simulink library "mbed_lib_hk"  (R2015a)
settings: Solver=ode45  SolverMode=SingleTasking  StartTime=0.0  StopTime=10.0  RelTol=1e-3
undefined symbols (not defined in the file): A
libraries: mbed_lib x1
(part 1 of 2)
settings Model: CovSFcnEnable=off  Creator=syoon  LastModifiedBy=Hendrik
settings OptimizationCC: BlockReduction=off  BooleanDataType=off
settings DebuggingCC: SaveWithParameterizedLinksMsg=none  UnderspecifiedInitializationDetection=Classic  MergeDetectMultiDrivingBlocksExec=none  SignalResolutionControl=TryResolveAllWithWarning  StrictBusMsg=Warning
settings HardwareCC: TargetUnknown=on

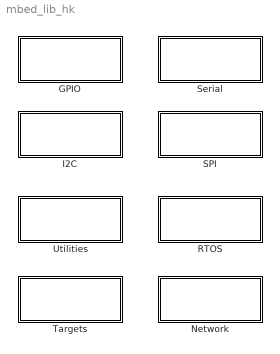
== system mbed_lib_hk ==
  GPIO : Subsystem
      mask Display: disp('GPIO')
  I2C : Subsystem
      mask Display: disp('I2C')
  Network : Subsystem
      mask Display: disp('Network')
  RTOS : Subsystem
      mask Display: disp('RTOS')
  SPI : Subsystem
      mask Display: disp('SPI')
  Serial : Subsystem
      mask Display: disp('Serial')
  Targets : Subsystem
      settings: OpenFcn=mbed_targets
      mask Display: disp('Targets')
  Utilities : Subsystem
      mask Display: disp('Utilities')

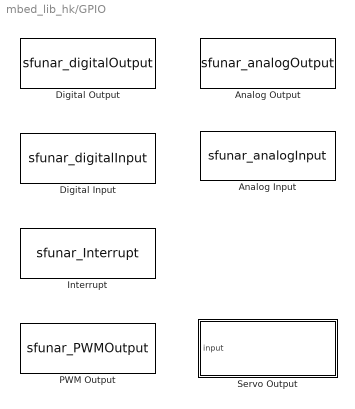
== system mbed_lib_hk/GPIO ==
  Analog Input : S-Function  FunctionName=sfunar_analogInput  Parameters=uint8(SParameter1), SampleTime, uint8(SParameter2)  mask(mbed Analog Input){SParameter2=A, SParameter1=0, SampleTime=-1}
      mask prompts: SParameter2 "Port Name:"; SParameter1 "Pin Number:"; SampleTime "Sample time (-1 for inherited):"
      mask help:
      | Reads the analog voltage input from the specified pin.
      |
      | The range of input on the pin is between 0 and Vref corresponding to a block output of 0 to 1.0f (in %) or 0 to 1024/4096/.. .
      mask Help:
      | <p>This block calls the AnalogIn.read() and AnalogIn.read_u16() function from the mbed library.
      | <p>For more information see: <a href="http://mbed.org ...">Arduino - AnalogRead</a>
      mask TypeOptions SParameter2: A | B | C | D | E | F | G | H | I | J | K
      mask TypeOptions SParameter1: 0 | 1 | 2 | 3 | 4 | 5 | 6 | 7 | 8 | 9 | 10 | 11 | 12 | 13 | 14 | 15
      mask Display:
      | offset=0.0;
      | plot([0+offset:0.025:0.25+offset],0.3*sin(2*pi*[0:0.1:1])+0.5)
      | disp(['Pin ', SParameter2+64, '.', num2str(SParameter1-1)]);
      | port_label('output',1,'RAW');
      | port_label('output',2,'0-1.0f');
  Analog Output : S-Function  FunctionName=sfunar_analogOutput  Parameters=uint8(SParameter1), SampleTime, uint8(SParameter2), uint8(inputVariant)  mask(mbed Analog Output){SParameter2=A, SParameter1=0, inputVariant=Double: 0 - 1.0f, SampleTime=-1}
      mask prompts: SParameter2 "Port Name:"; SParameter1 "Pin Number:"; inputVariant "Input data format"; SampleTime "Sample time (-1 for inherited):"
      mask help:
      | Writes an analog voltage output to the specified pin using the integrated DAC.
      |
      | The input to this block is a float between 0 and 1.0 (in %) or an integer between 0 and 1024/4096/.. corresponding to an output voltage between 0 to Vref.
      mask Help:
      | <p>This block calls the analogWrite() function from the Arduino language library.
      | <p>For more information see: <a href="http://arduino.cc/en/Reference/AnalogWrite">Arduino - AnalogWrite</a>
      mask TypeOptions SParameter2: A | B | C | D | E | F | G | H | I | J | K
      mask TypeOptions SParameter1: 0 | 1 | 2 | 3 | 4 | 5 | 6 | 7 | 8 | 9 | 10 | 11 | 12 | 13 | 14 | 15
      mask TypeOptions inputVariant: Uint16: RAW (0x0YYY) | Double: 0 - 1.0f
      mask Display:
      | offset=0.7;
      | plot([0+offset:0.025:0.25+offset],0.3*sin(2*pi*[0:0.1:1])+0.5)
      | disp(['Pin ', SParameter2+64, '.', num2str(SParameter1-1)]);
      | p={'RAW'; '0-1.0f'};
      | port_label('input',1,p{inputVariant});
  Digital Input : S-Function  FunctionName=sfunar_digitalInput  Parameters=uint8(SParameter1), SampleTime, uint8(SParameter2), uint8(SParameter3)  mask(mbed Digital Input){SParameter2=A, SParameter1=0, SParameter3=PullDefault, SampleTime=-1}
      mask prompts: SParameter2 "Port Name"; SParameter1 "Pin Number:"; SParameter3 "Input Mode"; SampleTime "Sample time (-1 for inherited):"
      mask help:
      | Reads the digital value from the specified pin.
      |
      | The block outputs 1 for high and 0 for low.
      mask Help:
      | <p>This block uses the DigitalIn api of the mbed library.
      | <p>For more information see: <a href="http://arduino.cc/en/Reference/DigitalRead">Arduino - DigitalRead</a>
      mask TypeOptions SParameter2: A | B | C | D | E | F | G | H | I | J | K
      mask TypeOptions SParameter1: 0 | 1 | 2 | 3 | 4 | 5 | 6 | 7 | 8 | 9 | 10 | 11 | 12 | 13 | 14 | 15
      mask TypeOptions SParameter3: PullDefault | PullUp | PullDown | PullNone
      mask Display:
      | plot([0 0.15 0.15 0.35 0.35 0.5],[0.3 0.3 0.7 0.7 0.3 0.3])
      | port_label('output',1,['Pin ', SParameter2+64, '.', num2str(SParameter1-1)]);
  Digital Output : S-Function  FunctionName=sfunar_digitalOutput  Parameters=uint8(SParameter1), SampleTime, uint8(SParameter2), uint8(SParameter3)  mask(mbed Digital Output){SParameter2=A, SParameter1=0, SParameter3=PullDefault, SampleTime=-1}
      mask prompts: SParameter2 "Port Name:"; SParameter1 "Pin Number:"; SParameter3 "Output Mode"; SampleTime "Sample time (-1 for inherited):"
      mask help:
      | Sends the digital value to the specified port.pin.
      | The pin can be configured as push-pull (pp) or open drain output (od).
      |
      | An input of 1 sets the pin high and 0 sets the pin low.
      mask Help:
      | <p>This block uses the DigitalOut class of the mbed library.
      | <p>For more information see: <a href="http://mbed.org">mbed - DigitalWrite</a>
      mask TypeOptions SParameter2: A | B | C | D | E | F | G | H | I | J | K
      mask TypeOptions SParameter1: 0 | 1 | 2 | 3 | 4 | 5 | 6 | 7 | 8 | 9 | 10 | 11 | 12 | 13 | 14 | 15
      mask TypeOptions SParameter3: PullDefault | PullUp | PullDown | PullNone | Repeater | OpenDrain
      mask Display:
      | plot([0.5 0.65 0.65 0.85 0.85 1],[0.3 0.3 0.7 0.7 0.3 0.3])
      | port_label('input',1,['Pin ', SParameter2+64, '.', num2str(SParameter1-1)]);
  Interrupt : S-Function  FunctionName=sfunar_Interrupt  Parameters=uint8(PortName), uint8(PinName), uint8(Interrupt)  mask{PortName=A, PinName=0, Interrupt=None}
      mask prompts: PortName "Port Name"; PinName "Pin Name"
      mask TypeOptions PortName: A | B | C | D | E | F | G | H | I | J | K
      mask TypeOptions PinName: 0 | 1 | 2 | 3 | 4 | 5 | 6 | 7 | 8 | 9 | 10 | 11 | 12 | 13 | 14 | 15
      mask TypeOptions Interrupt: None | Rise | Fall | Both
      mask Display:
      | p={'None'; 'Rise'; 'Fall'; 'Both'};
      | disp(['Interrupt: ' p{Interrupt} ' Pin ', PortName+64, '.', num2str(PinName-1)]);
  PWM Output : S-Function  FunctionName=sfunar_PWMOutput  Parameters=SampleTime, uint8(SParameter1), uint8(SParameter2), uint32(SParameter3)  mask(mbed PWM Output){SParameter1=A, SParameter2=0, SParameter3=1000, SampleTime=-1}
      mask prompts: SParameter1 "PWM Port:"; SParameter2 "PWM Pin:"; SParameter3 "Period (µs):"; SampleTime "Sample time (-1 for inherited):"
      mask help:
      | Creates an pwm output signal on the specified pin using a configurable PWM period.
      |
      | The input to this block is a float between 0.0f and 1.0f corresponding to 0 to 100% pulsewidth.
      mask Help:
      | <p>This block calls the analogWrite() function from the Arduino language library.
      | <p>For more information see: <a href="http://arduino.cc/en/Reference/AnalogWrite">Arduino - AnalogWrite</a>
      mask TypeOptions SParameter1: A | B | C | D | E | F | G | H | I | J | K
      mask TypeOptions SParameter2: 0 | 1 | 2 | 3 | 4 | 5 | 6 | 7 | 8 | 9 | 10 | 11 | 12 | 13 | 14 | 15
      mask Display:
      | plot([0.5 0.65 0.65 0.85 ],[0.3 0.3 0.7 0.7 ])
      | plot([0.8 0.8],[0.7 0.3])
      | plot([0.825 0.825],[0.7 0.3])
      | plot([0.85 0.85],[0.7 0.3])
      | plot([0.8 1],[0.3 0.3])
      | disp(['Pin ' SParameter1+64 '.' num2str(SParameter2-1)]);
      | port_label('input',1,'0-1.0f');
  Servo Output : Subsystem  mask{SParameter1=A, SParameter2=0, PW_min=1, PW_max=2}
      mask prompts: SParameter1 "PWM Port:"; SParameter2 "PWM Pin:"; PW_min "PW min (ms)"; PW_max "PW max (ms)"
      mask help:
      | Block generates PWM signal with 50Hz period for control of standard RC-servo.
      | Minimum and maximum pulsewidth can be configured.
      | Input is a double value between 0 and 1.0
      mask TypeOptions SParameter1: PWM Output/SParameter1
      mask TypeOptions SParameter2: PWM Output/SParameter2
      mask Display:
      | disp('Servo Output\n');
      | disp(['\nPin ' SParameter1+64 '.' num2str(SParameter2-1) ]);
      | port_label('input',1,'0-1.0f');

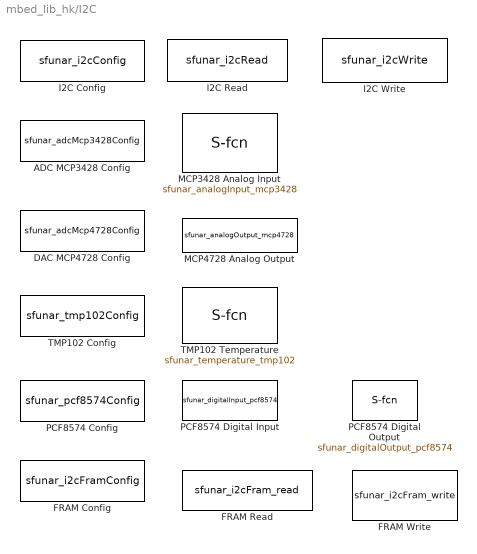
== system mbed_lib_hk/I2C ==
  ADC MCP3428 Config : S-Function  Priority=1  FunctionName=sfunar_adcMcp3428Config  Parameters=uint8(SParameter1)  mask(MCP3428 Configuration){SParameter1=0}
      mask prompts: SParameter1 "Device Sub Address"
      mask help:
      | This blocks sets up the MCP3428 on the I2C board. You must have one of these blocks in any model that ues this device.
      |
      | The sub-address must match the pin configuration on the board. See the board documentation for details.
      mask Display: disp(['Sub-Address: ' num2str(SParameter1) ]);
  DAC MCP4728 Config : S-Function  Priority=1  FunctionName=sfunar_adcMcp4728Config  Parameters=uint8(SParameter1)  mask(MCP4728 Configuration){SParameter1=0}
      mask prompts: SParameter1 "Device Sub Address"
      mask help:
      | This blocks sets up the MCP4728 on the I2C board. You must have one of these blocks in any model that ues this device.
      |
      | The sub-address must match the pin configuration on the board. See the board documentation for details.
      mask Display: disp(['Sub-Address: ' num2str(SParameter1) ]);
  FRAM Config : S-Function  Priority=1  FunctionName=sfunar_i2cFramConfig  mask(I2C Fram Config){}
  FRAM Read : S-Function  FunctionName=sfunar_i2cFram_read  Parameters=uint8(SParameter1-1), SampleTime, boolean(errEn)  mask(Fram Read){SampleTime=-1, SParameter1=on startup, errEn=on}
      mask prompts: SampleTime "Sample time (-1 for inherited):"; SParameter1 "Read condition"; errEn "Enable error output port"
      mask help: Reads one byte from the FRAM.
      mask TypeOptions SParameter1: on startup | on each step
      mask Display:
      | port_label('input', 1, 'Page Address');
      | port_label('input', 2, 'Word Address');
      | 
      | port_label('output',1,'Value');
      | if errEn
      | port_label('output',2,'Error');
      | end
  FRAM Write : S-Function  FunctionName=sfunar_i2cFram_write  Parameters=uint8(SParameter1-1), SampleTime, boolean(errEn)  mask(FRAM Write){SampleTime=-1, SParameter1=on startup, errEn=on}
      mask prompts: SampleTime "Sample time (-1 for inherited):"; SParameter1 "Write condition"; errEn "Enable error output port"
      mask help: Writes one byte to the FRAM
      mask TypeOptions SParameter1: on startup | on each step
      mask Display:
      | port_label('input', 1, 'Page Address');
      | port_label('input', 2, 'Word Address');
      | port_label('input', 3, 'Data');
      | 
      | if errEn
      | port_label('output',1,'Error');
      | end
  I2C Config : S-Function  Priority=0  FunctionName=sfunar_i2cConfig  Parameters=uint8(0), uint8(SParameter2), uint8(SParameter3), uint8(SParameter4), uint8(SParameter5), SParameter6, uint8(I2cPort)  mask(I2C Configuration){I2cPort=1, SParameter6=100000, SParameter2=B, SParameter3=9, SParameter4=B, SParameter5=8}
      mask prompts: I2cPort "I2C Port"; SParameter6 "Bus frequency: [Hz]"; SParameter2 "Port Name (SDA)"; SParameter3 "Pin Number (1-16):"; SParameter4 "Port Name (SCL)"; SParameter5 "Pin Number (1-16):"
      mask help: This blocks sets up the I2C connection on the mbed board. You must have one of these blocks in any model that ues I2C blocks.
      mask TypeOptions I2cPort: 1 | 2 | 3
      mask TypeOptions SParameter2: A | B | C | D | E | F
      mask TypeOptions SParameter3: 0 | 1 | 2 | 3 | 4 | 5 | 6 | 7 | 8 | 9 | 10 | 11 | 12 | 13 | 14 | 15
      mask TypeOptions SParameter4: A | B | C | D | E | F
      mask TypeOptions SParameter5: 0 | 1 | 2 | 3 | 4 | 5 | 6 | 7 | 8 | 9 | 10 | 11 | 12 | 13 | 14 | 15
      mask Display:
      | disp(['I2C ' num2str(I2cPort) '\n\n']);
      | disp(['SDA: ' SParameter2+64 '.' num2str(SParameter3-1) ', SCL: ' SParameter4+64, '.' num2str(SParameter5-1)]);
      | disp(['\n\nFrequency: ' num2str(SParameter6) ' HZ']);
  I2C Read : S-Function  FunctionName=sfunar_i2cRead  Parameters=SampleTime, boolean(AddressFlag), uint8(SlaveAddress), boolean(ByteCountFlag), uint8(NumBytes), boolean(Repeated), uint8(I2cPort)  mask{I2cPort=1, AddressFlag=off, SlaveAddress=0, ByteCountFlag=off, NumBytes=1, Repeated=off, SampleTime=-1}
      mask prompts: I2cPort "I2C Port:"; AddressFlag "external address input"; SlaveAddress "Slave address (7 bit):"; ByteCountFlag "external byte count"; NumBytes "Number of bytes to read:"; SampleTime "Sample time (-1 for inherited):"
      mask TypeOptions I2cPort: 1 | 2 | 3
      mask Display:
      | disp(['I2C ' num2str(I2cPort) '\n']);
      | if AddressFlag == 0
      |     disp(['\nAddress: 0x' dec2hex(SlaveAddress)]);
      | else
      |    disp(['\nAddress: external']);
      |    port_label('input',1,'addr');
      | end
      | 
      | if ByteCountFlag == 1 && AddressFlag == 0
      |     port_label('input',1,'cnt');
      | elseif ByteCountFlag == 1 && AddressFlag == 1
      |     port_label('input',2,'cnt');
      | end
  I2C Write : S-Function  FunctionName=sfunar_i2cWrite  Parameters=SampleTime, boolean(AddressFlag), uint8(SlaveAddress), boolean(ByteCountFlag), boolean(Repeated), uint8(I2cPort)  mask{I2cPort=1, AddressFlag=off, SlaveAddress=0, ByteCountFlag=off, Repeated=off, SampleTime=-1}
      mask prompts: I2cPort "I2C Port:"; AddressFlag "external address input"; SlaveAddress "Slave address (7bit):"; ByteCountFlag "external byte count"; SampleTime "Sample time (-1 for inherited):"
      mask TypeOptions I2cPort: 1 | 2 | 3
      mask Display:
      | disp(['I2C ' num2str(I2cPort) '\n']);
      | 
      | port_label('input', 1, 'data');
      | 
      | if AddressFlag == 1
      |     disp(['\nAddress: external']);
      |     port_label('input', 2, 'addr');
      | else
      |     disp(['\nAddress: 0x' dec2hex(SlaveAddress)]);
      | end
      | 
      | if AddressFlag == 0 && ByteCountFlag == 1
      |     port_label('input', 2, 'cnt');
      | elseif AddressFlag == 1 && ByteCountFlag == 1
      |     port_label('input', 3, 'cnt');
      | end
  MCP3428 Analog Input : S-Function  FunctionName=sfunar_analogInput_mcp3428  Parameters=uint8(SParameter1-1), SampleTime, uint8(SParameter2), uint8(SParameter3), boolean(ErrorOutputEnable)  mask(MCP3428 Analog Input){SampleTime=-1, SParameter1=0, SParameter2=240 SPS (12 bit), SParameter3=1X, ErrorOutputEnable=on}
      mask prompts: SampleTime "Sample time (-1 for inherited):"; SParameter1 "Pin Number:"; SParameter2 "Sample-Rate"; SParameter3 "PGA-Gain"; ErrorOutputEnable "Enable error output port"
      mask help:
      | Reads the analog voltage input from the specified pin on the MCP3428.
      |
      | Warning: This block waits for a complete conversation during the execution step.
      | If the sample time is too small it will have an impact on the step time of the whole model!
      mask TypeOptions SParameter1: 0 | 1 | 2 | 3 | 4 | 5 | 6 | 7
      mask TypeOptions SParameter2: 240 SPS (12 bit) | 60 SPS (14 bit) | 15 SPS (16 bit)
      mask TypeOptions SParameter3: 1X | 2X | 4X | 8X
      mask Display:
      | plot([0:0.01:0.25],0.3*sin(2*pi*[0:0.04:1])+0.5)
      | disp(['Pin ', num2str(SParameter1-1)]);
      | port_label('output',1,'RAW');
      | port_label('output',2,'V');
      | port_label('output',3,'0-1');
      | if ErrorOutputEnable
      |     port_label('output',4,'Error');
      | end
  MCP4728 Analog Output : S-Function  FunctionName=sfunar_analogOutput_mcp4728  Parameters=uint8(SParameter1-1), SampleTime, boolean(errEn), uint8(inputVariant-1), boolean(internalRef-1), boolean(gain2x-1)  mask(MCP4728 Analog Output){SampleTime=-1, SParameter1=0, inputVariant=Uint16: right aligned (0x0YYY), internalRef=VDD (3.3 V), gain2x=1X, errEn=on}
      mask prompts: SampleTime "Sample time (-1 for inherited):"; SParameter1 "Pin Number:"; inputVariant "Input data format"; internalRef "Reference voltage"; gain2x "Gain"; errEn "Enable error output port"
      mask help: Approximates an analog output on the specified pin on the MCP4728.
      mask TypeOptions SParameter1: 0 | 1 | 2 | 3
      mask TypeOptions inputVariant: Uint16: right aligned (0x0YYY) | Uint16: left aligned (0xYYY0) | Double: Voltage in V | Double: 0 ... 1
      mask TypeOptions internalRef: VDD (3.3 V) | Internal (2.048 V)
      mask TypeOptions gain2x: 1X | 2X (only for internal VRef)
      mask Display:
      | plot([0.5-.125:0.01:0.75-.125],0.3*sin(2*pi*[0:0.04:1])+0.5)
      | port_label('input',1,['Pin ', num2str(SParameter1-1)]);
      | if errEn
      |     port_label('output',1,'Error');
      | end
  PCF8574 Config : S-Function  Priority=1  FunctionName=sfunar_pcf8574Config  Parameters=uint8(SParameter1)  mask(PCF8574 Configuration){SParameter1=0}
      mask prompts: SParameter1 "Device Sub Address"
      mask help:
      | This blocks sets up the PCF8574 on the I2C board. You must have one of these blocks in any model that ues this device.
      |
      | The sub-address must match the pin configuration on the board. See the board documentation for details.
      mask Display: disp(['Sub-Address: ' num2str(SParameter1) ]);
  PCF8574 Digital Input : S-Function  FunctionName=sfunar_digitalInput_pcf8574  Parameters=uint8(SParameter1-1), SampleTime, boolean(errEn)  mask(PCF8574 Digital Input){SampleTime=-1, SParameter1=0, errEn=on}
      mask prompts: SampleTime "Sample time (-1 for inherited):"; SParameter1 "Pin Number:"; errEn "Enable error output port"
      mask help:
      | Reads the digital value from the specified pin of the PCF8574.
      |
      | Note: The PCF8574 has an pull up current source on each pin.
      mask TypeOptions SParameter1: 0 | 1 | 2 | 3 | 4 | 5 | 6 | 7
      mask Display:
      | disp(['Pin ', num2str(SParameter1-1)]);
      | port_label('output',1,'Value');
      | if errEn
      | port_label('output',2,'Error');
      | end
  PCF8574 Digital Output : S-Function  FunctionName=sfunar_digitalOutput_pcf8574  Parameters=uint8(SParameter1-1), SampleTime, boolean(errEn)  mask(PCF8574 digital output){SampleTime=-1, SParameter1=0, errEn=on}
      mask prompts: SampleTime "Sample time (-1 for inherited):"; SParameter1 "Pin Number:"; errEn "Enable error output port"
      mask help:
      | Set an digital pin of the PCF8574.
      |
      | Note: The PCF8574 has a high level output current of max. 300 µA but it can sink up to 25 mA on a low level output.
      mask TypeOptions SParameter1: 0 | 1 | 2 | 3 | 4 | 5 | 6 | 7
      mask Display:
      | port_label('input',1,['Pin ', num2str(SParameter1-1)]);
      | if errEn
      | port_label('output',1,'Error');
      | end
  TMP102 Config : S-Function  Priority=1  FunctionName=sfunar_tmp102Config  Parameters=uint8(SParameter1), uint8(SParameter2)  mask(TMP102 Configuration){SParameter1=0, SParameter2=4 Hz}
      mask prompts: SParameter1 "Device Sub Address"; SParameter2 "Samplerate"
      mask help:
      | This blocks sets up the TMP102 on the I2C board. You must have one of these blocks in any model that ues this device.
      |
      | The sub-address must match the pin configuration on the board. See the board documentation for details.
      mask TypeOptions SParameter2: 0.25 Hz | 1 Hz | 4 Hz | 8 Hz
      mask Display: disp(['Sub-Address: ' num2str(SParameter1) ]);
  TMP102 Temperature : S-Function  FunctionName=sfunar_temperature_tmp102  Parameters=uint8(0), SampleTime, boolean(errEn)  mask(TMP102 Temperature Input){SampleTime=-1, errEn=on}
      mask prompts: SampleTime "Sample time (-1 for inherited):"; errEn "Enable error output port"
      mask help:
      | Reads the last conversation result of the TMP102.
      |
      | Warning: The TMP102 needs at least 26 ms for one conversation.
      | If the sample time for this block is faster than this time the sensor may not produce valid values.
      mask Display:
      | disp(['Temperature']);
      | port_label('output',1,'RAW');
      | port_label('output',2,'°C');
      | if errEn
      | port_label('output',3,'Error');
      | end

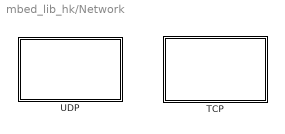
== system mbed_lib_hk/Network ==
  TCP : Subsystem
      mask Display: disp('TCP')
  UDP : Subsystem
      mask Display: disp('UDP')

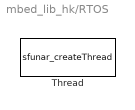
== system mbed_lib_hk/RTOS ==
  Thread : S-Function  FunctionName=sfunar_createThread  Parameters=ThreadPriority, StackOption, uint32(StackSize), uint32(Timing)  mask{ThreadPriority=Normal, Timing=0, StackOption=Default, StackSize=0}
      mask prompts: ThreadPriority "Thread Priority"; StackOption "Stack size"; StackSize "Size:"
      mask TypeOptions ThreadPriority: Idle | Low | Below Normal | Normal | Above Normal | High | Realtime
      mask TypeOptions StackOption: Default | User defined
      mask Display: disp('create RtosThread');

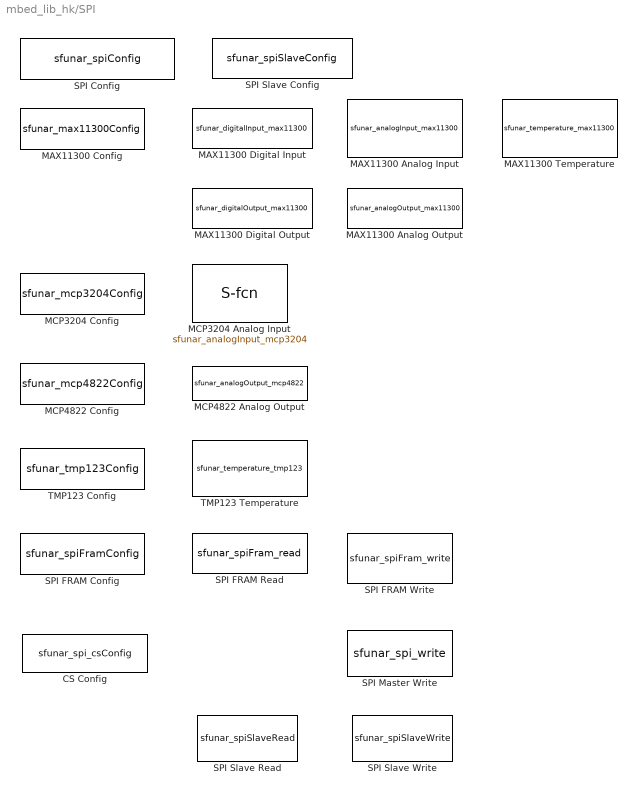
== system mbed_lib_hk/SPI ==
  CS Config : S-Function  FunctionName=sfunar_spi_csConfig  Parameters=CS_PORT, CS_PIN  mask{CS_PORT=A, CS_PIN=0}
      mask prompts: CS_PORT "Chip select: Port"; CS_PIN "Pin"
      mask TypeOptions CS_PORT: A | B | C | D
      mask TypeOptions CS_PIN: 0 | 1 | 2 | 3 | 4 | 5 | 6 | 7 | 8 | 9 | 10 | 11 | 12 | 13 | 14 | 15
      mask Display: disp(['Chip Select: ' CS_PORT+64, '.' num2str(CS_PIN-1)]);
  MAX11300 Analog Input : S-Function  FunctionName=sfunar_analogInput_max11300  Parameters=mode-1, SampleTime, posPin-1, negPin-1, power-1, range-1, ref-1, boolean(ErrorOutputEnable)  mask(MAX11300 Analog Input){SampleTime=-1, mode=Single-Ended, posPin=1, negPin=1, power=1, range=0 to +10, ref=Internal (2.5 V), ErrorOutputEnable=on}
      mask prompts: SampleTime "Sample time (-1 for inherited):"; posPin "positive input pin"; negPin "negative input pin"; power "Average samples"; ref "Reference voltage"; ErrorOutputEnable "Enable error output"
      mask help: Reads the analog voltage input from the specified pin on the MAX11300.
      mask TypeOptions mode: Single-Ended | Differential
      mask TypeOptions posPin: 0 | 1 | 2 | 3 | 4 | 5 | 6 | 7 | 8 | 9 | 10 | 11 | 12 | 13 | 14 | 15 | 16 | 17 | 18 | 19
      mask TypeOptions negPin: 0 | 1 | 2 | 3 | 4 | 5 | 6 | 7 | 8 | 9 | 10 | 11 | 12 | 13 | 14 | 15 | 16 | 17 | 18 | 19
      mask TypeOptions power: 1 | 2 | 4 | 8 | 16 | 32 | 64 | 128
      mask TypeOptions range: Non selected | 0 to +10 | -5 to +5 | -10 to 0 | 0 to +2.5 | --- | 0 to +2.5 | ---
      mask TypeOptions ref: Internal (2.5 V) | External
      mask Display:
      | plot([0:0.01:0.25],0.3*sin(2*pi*[0:0.04:1])+0.5)
      | %disp(['Pin ', num2str(SParameter1-1)]);
      | port_label('output',1,'RAW');
      | port_label('output',2,'0-1');
      | if ErrorOutputEnable
      |     port_label('output',3,'Error');
      | end
  MAX11300 Analog Output : S-Function  FunctionName=sfunar_analogOutput_max11300  Parameters=pin-1, SampleTime, boolean(errEn), uint8(inputVariant-1), range-1  mask(MAX11300 Analog Output){SampleTime=-1, pin=0, inputVariant=Uint16: left aligned (0x0YYY), range=0 to +10 V, errEn=on}
      mask prompts: SampleTime "Sample time (-1 for inherited):"; pin "Pin Number:"; inputVariant "Input data format"; errEn "Enable error output port"
      mask help:
      | Approximates an analog output on the specified pin on the MAX11300.
      |
      | Note: It can take up to 1 ms before the output voltage is updated on the pin.
      mask TypeOptions pin: 0 | 1 | 2 | 3 | 4 | 5 | 6 | 7 | 8 | 9 | 10 | 11 | 12 | 13 | 14 | 15 | 16 | 17 | 18 | 19
      mask TypeOptions inputVariant: Uint16: left aligned (0x0YYY) | Uint16: right aligned (0xYYY0) | Double: 0 ... 1
      mask TypeOptions range: Non selected | 0 to +10 V | -5 to +5  | -10 to 0  | -5 to +5 | --- | 0 to +10 | ---
      mask Display:
      | plot([0.5-.125:0.01:0.75-.125],0.3*sin(2*pi*[0:0.04:1])+0.5)
      | port_label('input',1,['Pin ', num2str(pin-1)]);
      | if errEn
      |     port_label('output',1,'Error');
      | end
  MAX11300 Config : S-Function  Priority=1  FunctionName=sfunar_max11300Config  Parameters=CS_PORT, CS_PIN, ADCCONV-1, DACREF-1  mask(MAX11300 Configuration){CS_PORT=B, CS_PIN=6, ADCCONV=200 kSPS, DACREF=Internal (2.5 V)}
      mask prompts: CS_PORT "Chip Select: Port"; CS_PIN "Pin"; ADCCONV "ADC Conversion Rate"; DACREF "DAC Reference"
      mask help: This blocks sets up the MAX11300. You must have one of these blocks in any model that ues this device.
      mask TypeOptions CS_PORT: A | B | C | D | E | F
      mask TypeOptions CS_PIN: 0 | 1 | 2 | 3 | 4 | 5 | 6 | 7 | 8 | 9 | 10 | 11 | 12 | 13 | 14 | 15
      mask TypeOptions ADCCONV: 200 kSPS | 250 kSPS | 333 kSPS | 400 kSPS
      mask TypeOptions DACREF: External | Internal (2.5 V)
      mask Display: disp(['Chip Select: ' CS_PORT+64, '.' num2str(CS_PIN-1)]);
  MAX11300 Digital Input : S-Function  FunctionName=sfunar_digitalInput_max11300  Parameters=pin-1, SampleTime, boolean(errEn), thres  mask(MAX11300 Digital Input){SampleTime=-1, pin=0, thres=1638, errEn=on}
      mask prompts: SampleTime "Sample time (-1 for inherited):"; pin "Pin Number:"; thres "Threshold:"; errEn "Enable error output port"
      mask help:
      | Reads the digital value from the specified pin of the MAX11300.
      |
      | Note: The external voltage is compared to an internal reference which can be
      | controlled by the threshold.
      | The threshold must be a number between 0 and 4095 (2^12-1) corresponding to a voltage of 0 to 5 V.
      mask TypeOptions pin: 0 | 1 | 2 | 3 | 4 | 5 | 6 | 7 | 8 | 9 | 10 | 11 | 12 | 13 | 14 | 15 | 16 | 17 | 18 | 19
      mask Display:
      | port_label('output',1,['Pin ', num2str(pin-1), ' > ', num2str(thres*5/(2^12-1)), ' V']);
      | if errEn
      | port_label('output',2,'Error');
      | end
  MAX11300 Digital Output : S-Function  FunctionName=sfunar_digitalOutput_max11300  Parameters=pin-1, SampleTime, boolean(errEn), level  mask(MAX11300 digital output){SampleTime=-1, pin=0, level=2^12-1, errEn=on}
      mask prompts: SampleTime "Sample time (-1 for inherited):"; pin "Pin Number:"; level "Output level:"; errEn "Enable error output port"
      mask help:
      | Set an digital pin of the MAX11300.
      |
      | Note: The external voltage is set to an internal reference which can be
      | controlled by the level.
      | The level must be a number between 0 and 4095 (2^12-1) corresponding to a voltage of 0 to 5 V.
      mask TypeOptions pin: 0 | 1 | 2 | 3 | 4 | 5 | 6 | 7 | 8 | 9 | 10 | 11 | 12 | 13 | 14 | 15 | 16 | 17 | 18 | 19
      mask Display:
      | disp(['H-Level = ', num2str(level*5/(2^12-1)), ' V']);
      | port_label('input',1,['Pin ', num2str(pin-1)]);
      | if errEn
      | port_label('output',1,'Error');
      | end
  MAX11300 Temperature : S-Function  FunctionName=sfunar_temperature_max11300  Parameters=chan, SampleTime, boolean(errEn)  mask(MAX11300 Temperature Input){SampleTime=-1, chan=Internal, errEn=on}
      mask prompts: SampleTime "Sample time (-1 for inherited):"; chan "Channel"; errEn "Enable error output port"
      mask help: Reads the last conversation result of the MAX11300.
      mask TypeOptions chan: Internal | External 1 | External 2
      mask Display:
      | disp(['Temperature\nChannel: ' int2str(chan-1)]);
      | port_label('output',1,'RAW');
      | port_label('output',2,'°C');
      | if errEn
      | port_label('output',3,'Error');
      | end
  MCP3204 Analog Input : S-Function  FunctionName=sfunar_analogInput_mcp3204  Parameters=mode-1, SampleTime, pin-1, boolean(ErrorOutputEnable)  mask(MCP3204 Analog Input){SampleTime=-1, mode=Single-Ended, pin=1, ErrorOutputEnable=on}
      mask prompts: SampleTime "Sample time (-1 for inherited):"; ErrorOutputEnable "Enable error output"
      mask help: Reads the analog voltage input from the specified pin on the MCP3204.
      mask TypeOptions mode: Differential | Single-Ended
      mask TypeOptions pin: 0 | 1 | 2 | 3
      mask Display:
      | plot([0:0.01:0.25],0.3*sin(2*pi*[0:0.04:1])+0.5)
      | %disp(['Pin ', num2str(SParameter1-1)]);
      | port_label('output',1,'RAW');
      | port_label('output',2,'0-1');
      | if ErrorOutputEnable
      |     port_label('output',3,'Error');
      | end
  MCP3204 Config : S-Function  Priority=1  FunctionName=sfunar_mcp3204Config  Parameters=CS_PORT, CS_PIN  mask(MCP3204 Configuration){CS_PORT=B, CS_PIN=6}
      mask prompts: CS_PORT "Chip Select: Port"; CS_PIN "Pin"
      mask help: This blocks sets up the MCP3204. You must have one of these blocks in any model that ues this device.
      mask TypeOptions CS_PORT: A | B | C | D | E | F
      mask TypeOptions CS_PIN: 0 | 1 | 2 | 3 | 4 | 5 | 6 | 7 | 8 | 9 | 10 | 11 | 12 | 13 | 14 | 15
      mask Display: disp(['Chip Select: ' CS_PORT+64, '.' num2str(CS_PIN-1)]);
  MCP4822 Analog Output : S-Function  FunctionName=sfunar_analogOutput_mcp4822  Parameters=pin-1, SampleTime, boolean(errEn), uint8(inputVariant-1), gain-1  mask(MCP4822 Analog Output){SampleTime=-1, pin=0, inputVariant=Uint16: right aligned (0x0YYY), gain=1X, errEn=on}
      mask prompts: SampleTime "Sample time (-1 for inherited):"; pin "Pin Number:"; inputVariant "Input data format"; errEn "Enable error output port"
      mask help: Approximates an analog output on the specified pin on the MCP4822.
      mask TypeOptions pin: 0 | 1
      mask TypeOptions inputVariant: Uint16: right aligned (0x0YYY) | Uint16: left aligned (0xYYY0) | Double: 0 ... 1
      mask TypeOptions gain: 2X | 1X
      mask Display:
      | plot([0.5-.125:0.01:0.75-.125],0.3*sin(2*pi*[0:0.04:1])+0.5)
      | port_label('input',1,['Pin ', num2str(pin-1)]);
      | if errEn
      |     port_label('output',1,'Error');
      | end
  MCP4822 Config : S-Function  Priority=1  FunctionName=sfunar_mcp4822Config  Parameters=CS_PORT, CS_PIN  mask(MCP4822 Configuration){CS_PORT=B, CS_PIN=6}
      mask prompts: CS_PORT "Chip Select: Port"; CS_PIN "Pin"
      mask help: This blocks sets up the MCP4822. You must have one of these blocks in any model that ues this device.
      mask TypeOptions CS_PORT: A | B | C | D | E | F
      mask TypeOptions CS_PIN: 0 | 1 | 2 | 3 | 4 | 5 | 6 | 7 | 8 | 9 | 10 | 11 | 12 | 13 | 14 | 15
      mask Display: disp(['Chip Select: ' CS_PORT+64, '.' num2str(CS_PIN-1)]);
  SPI Config : S-Function  Priority=0  FunctionName=sfunar_spiConfig  Parameters=uint8(0), uint8(SParameter2), uint8(SParameter3), uint8(SParameter4), uint8(SParameter5), SParameter6, uint8(SCK_PORT), uint8(SCK_PIN)  mask(SPI Configuration){SParameter6=100000, SParameter2=A, SParameter3=7, SParameter4=A, SParameter5=6, SCK_PORT=A, SCK_PIN=5}
      mask prompts: SParameter6 "Bus frequency: [Hz]"; SParameter2 "MOSI: Port"; SParameter3 "Pin"; SParameter4 "MISO: Port"; SParameter5 "Pin"; SCK_PORT "SCK: Port"; SCK_PIN "Pin"
      mask help: This blocks sets up the SPI connection on the mbed board. You must have one of these blocks in any model that ues SPI blocks.
      mask TypeOptions SParameter2: A | B | C | D | E | F
      mask TypeOptions SParameter3: 0 | 1 | 2 | 3 | 4 | 5 | 6 | 7 | 8 | 9 | 10 | 11 | 12 | 13 | 14 | 15
      mask TypeOptions SParameter4: A | B | C | D | E | F
      mask TypeOptions SParameter5: 0 | 1 | 2 | 3 | 4 | 5 | 6 | 7 | 8 | 9 | 10 | 11 | 12 | 13 | 14 | 15
      mask TypeOptions SCK_PORT: A | B | C | D | E | F
      mask TypeOptions SCK_PIN: 0 | 1 | 2 | 3 | 4 | 5 | 6 | 7 | 8 | 9 | 10 | 11 | 12 | 13 | 14 | 15
      mask Display:
      | disp(['MOSI: ' SParameter2+64 '.' num2str(SParameter3-1) ', MISO: ' SParameter4+64, '.' num2str(SParameter5-1)  ', SCK: ' SCK_PORT+64, '.' num2str(SCK_PIN-1) ' \n']);
      | disp(['\nFrequency: ' num2str(SParameter6) ' HZ']);
  SPI FRAM Config : S-Function  Priority=1  FunctionName=sfunar_spiFramConfig  Parameters=CS_PORT, CS_PIN  mask(SPI FRAM Configuration){CS_PORT=B, CS_PIN=6}
      mask prompts: CS_PORT "Chip Select: Port"; CS_PIN "Pin"
      mask help: This blocks sets up the FRAM. You must have one of these blocks in any model that ues this device.
      mask TypeOptions CS_PORT: A | B | C | D | E | F
      mask TypeOptions CS_PIN: 0 | 1 | 2 | 3 | 4 | 5 | 6 | 7 | 8 | 9 | 10 | 11 | 12 | 13 | 14 | 15
      mask Display: disp(['Chip Select: ' CS_PORT+64, '.' num2str(CS_PIN-1)]);
  SPI FRAM Read : S-Function  FunctionName=sfunar_spiFram_read  Parameters=uint8(SParameter1-1), SampleTime, boolean(errEn)  mask(FRAM Read){SampleTime=-1, SParameter1=on startup, errEn=on}
      mask prompts: SampleTime "Sample time (-1 for inherited):"; SParameter1 "Read condition"; errEn "Enable error output port"
      mask help: Reads one byte from the FRAM
      mask TypeOptions SParameter1: on startup | on each step
      mask Display:
      | port_label('input', 1, 'Page Address');
      | port_label('input', 2, 'Word Address');
      | 
      | port_label('output',1,'Value');
      | if errEn
      | port_label('output',2,'Error');
      | end
  SPI FRAM Write : S-Function  FunctionName=sfunar_spiFram_write  Parameters=uint8(SParameter1-1), SampleTime, boolean(errEn)  mask(FRAM write){SampleTime=-1, SParameter1=on startup, errEn=on}
      mask prompts: SampleTime "Sample time (-1 for inherited):"; SParameter1 "Write condition"; errEn "Enable error output port"
      mask help: Writes one byte to the FRAM
      mask TypeOptions SParameter1: on startup | on each step
      mask Display:
      | port_label('input', 1, 'Page Address');
      | port_label('input', 2, 'Word Address');
      | port_label('input', 3, 'Data');
      | 
      | if errEn
      | port_label('output',1,'Error');
      | end
  SPI Master Write : S-Function  FunctionName=sfunar_spi_write  Parameters=SampleTime  mask{SampleTime=-1}
      mask prompts: SampleTime "Sample time (-1 for inherited):"
      mask Display: disp('SPI Master Write');
  SPI Slave Config : S-Function  FunctionName=sfunar_spiSlaveConfig  Parameters=BusSpeed, MosiPort, MosiPin, MisoPort, MisoPin, SckPort, SckPin, SselPort, SselPin  mask{BusSpeed=100000, MosiPort=A, MosiPin=0, MisoPort=A, MisoPin=0, SckPort=A, SckPin=0, SselPort=A, SselPin=0}
      mask prompts: BusSpeed "Bus frequency: [Hz]"; MosiPort "MOSI: Port"; MosiPin "Pin"; MisoPort "MISO: Port"; MisoPin "Pin"; SckPort "SCK: Port"; SckPin "Pin"; SselPort "SSEL: Port"; SselPin "Pin"
      mask TypeOptions MosiPort: A | B | C | D | E | F
      mask TypeOptions MosiPin: 0 | 1 | 2 | 3 | 4 | 5 | 6 | 7 | 8 | 9 | 10 | 11 | 12 | 13 | 14 | 15
      mask TypeOptions MisoPort: A | B | C | D | E | F
      mask TypeOptions MisoPin: 0 | 1 | 2 | 3 | 4 | 5 | 6 | 7 | 8 | 9 | 10 | 11 | 12 | 13 | 14 | 15
      mask TypeOptions SckPort: A | B | C | D | E | F
      mask TypeOptions SckPin: 0 | 1 | 2 | 3 | 4 | 5 | 6 | 7 | 8 | 9 | 10 | 11 | 12 | 13 | 14 | 15
      mask TypeOptions SselPort: A | B | C | D | E | F
      mask TypeOptions SselPin: 0 | 1 | 2 | 3 | 4 | 5 | 6 | 7 | 8 | 9 | 10 | 11 | 12 | 13 | 14 | 15
      mask Display:
      | disp(['Frequency: ' num2str(BusSpeed) ' HZ\n\n']);
      | disp(['\nMOSI: ' MosiPort+64 '.' num2str(MosiPin-1) ', MISO: ' MisoPort+64, '.' num2str(MisoPin-1) '\n']);
      | disp(['\n\n\nSCK: ' SckPort+64, '.' num2str(SckPin-1) ',SSEL: ' SselPort+64 '.' num2str(SselPin-1) '\n']);
  SPI Slave Read : S-Function  FunctionName=sfunar_spiSlaveRead  Parameters=SampleTime  mask{SampleTime=-1}
      mask prompts: SampleTime "Sampel time: (-1 for inherited)"
      mask Display: disp('SPI Slave Read')
  SPI Slave Write : S-Function  FunctionName=sfunar_spiSlaveWrite  Parameters=SampleTime  mask{SampleTime=-1}
      mask prompts: SampleTime "Sample time: (-1 for inherited)"
      mask Display: disp('SPI Slave Write');
  TMP123 Config : S-Function  Priority=1  FunctionName=sfunar_tmp123Config  Parameters=CS_PORT, CS_PIN  mask(TMP123 Configuration){CS_PORT=B, CS_PIN=6}
      mask prompts: CS_PORT "Chip Select: Port"; CS_PIN "Pin"
      mask help: This blocks sets up the TMP123. You must have one of these blocks in any model that ues this device.
      mask TypeOptions CS_PORT: A | B | C | D | E | F
      mask TypeOptions CS_PIN: 0 | 1 | 2 | 3 | 4 | 5 | 6 | 7 | 8 | 9 | 10 | 11 | 12 | 13 | 14 | 15
      mask Display: disp(['Chip Select: ' CS_PORT+64, '.' num2str(CS_PIN-1)]);
  TMP123 Temperature : S-Function  FunctionName=sfunar_temperature_tmp123  Parameters=uint8(0), SampleTime, boolean(errEn)  mask(TMP123 Temperature Input){SampleTime=-1, errEn=on}
      mask prompts: SampleTime "Sample time (-1 for inherited):"; errEn "Enable error output port"
      mask help:
      | Reads the last conversation result of the TMP123.
      |
      | Warning: The TMP123 needs 320 ms max for one conversation.
      | If the sample time for this block is faster than this time the sensor may not produce valid values.
      mask Display:
      | disp(['Temperature']);
      | port_label('output',1,'RAW');
      | port_label('output',2,'°C');
      | if errEn
      | port_label('output',3,'Error');
      | end

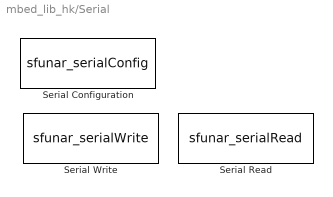
== system mbed_lib_hk/Serial ==
  Serial Configuration : S-Function  FunctionName=sfunar_serialConfig  Parameters=uint8(SerialPort), uint8(TXPort), uint8(TXPin), uint8(RXPort), uint8(RXPin), BaudRate  mask(Arduino Serial Configuration){SerialPort=1, TXPort=A, TXPin=2, RXPort=A, RXPin=3, BaudRate=9600}
      mask prompts: SerialPort "Serial Port"; TXPort "Port Name (TX)"; TXPin "Pin Number (1-16):"; RXPort "Port Name (RX)"; RXPin "Pin Number (1-16):"; BaudRate "Baud Rate:"
      mask help:
      | This blocks sets up the serial connection on the Arduino board. You must have one of these blocks in any model that ues the Serial Send or Serial Read blocks.
      |
      | Set the baud rate to match the device that you are communicating with. Standard rates include:300, 1200, 2400, 4800, 9600, 14400, 19200, 28800, 38400, 57600, or 115200.
      mask Help:
      | <p>This block calls the Serial.begin() function from the Arduino language library.
      | <p>For more information see: <a href="http://arduino.cc/en/Serial/Begin">Arduino - Serial/Begin</a>
      mask TypeOptions SerialPort: 1 | 2 | 3 | 4 | 5
      mask TypeOptions TXPort: A | B | C | D | E | F
      mask TypeOptions TXPin: 0 | 1 | 2 | 3 | 4 | 5 | 6 | 7 | 8 | 9 | 10 | 11 | 12 | 13 | 14 | 15
      mask TypeOptions RXPort: A | B | C | D | E | F
      mask TypeOptions RXPin: 0 | 1 | 2 | 3 | 4 | 5 | 6 | 7 | 8 | 9 | 10 | 11 | 12 | 13 | 14 | 15
      mask Display:
      | disp(['Serial' num2str(SerialPort) '\n\n']);
      | disp(['TX ' TXPort+64 '.' num2str(TXPin-1) ', RX ' RXPort+64, '.' num2str(RXPin-1)]);
  Serial Read : S-Function  FunctionName=sfunar_serialRead  Parameters=SampleTime, uint8(SParameter1)  mask(Arduino Serial Read){SParameter1=Serial1, SampleTime=-1}
      mask prompts: SParameter1 "Serial Port"; SampleTime "Sample time (-1 for inherited):"
      mask help:
      | Reads one byte from the serial interface on the Arduino board.
      |
      | Outputs -1 if no data is available to be read.
      mask Help:
      | <p>This block calls the Serial.read() function from the Arduino language library.
      | <p>For more information see: <a href="http://arduino.cc/en/Serial/Read">Arduino - Serial/Read</a>
      mask TypeOptions SParameter1: Serial1 | Serial2 | Serial3 | Serial4 | Serial5
      mask Display:
      | p={'Serial1'; 'Serial2'; 'Serial3'; 'Serial4'; 'Serial5'};
      | disp([p{SParameter1} ' Read'])
  Serial Write : S-Function  FunctionName=sfunar_serialWrite  Parameters=SampleTime, uint8(SParameter1)  mask(Arduino Serial Write){SParameter1=Serial1, SampleTime=-1}
      mask prompts: SParameter1 "Serial Port"; SampleTime "Sample time (-1 for inherited):"
      mask help:
      | Writes a vector of bytes to the serial port on the Arduino board.
      |
      | Outputs -1 if no data is available to be read.
      mask Help:
      | <p>This block calls the Serial.write() function from the Arduino language library.
      | <p>For more information see: <a href="http://arduino.cc/en/Serial/Write">Arduino - Serial/Write</a>
      mask TypeOptions SParameter1: Serial1 | Serial2 | Serial3 | Serial4 | Serial5
      mask Display:
      | p={'Serial1'; 'Serial2'; 'Serial3'; 'Serial4'; 'Serial5'};
      | disp([p{SParameter1} ' Write'])

== system mbed_lib_hk/Targets ==

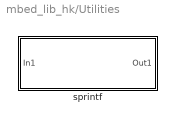
== system mbed_lib_hk/Utilities ==
  sprintf : Subsystem  mask{format=%f\r\n}
      mask TypeOptions format: %f\r\n | %d\r\n | %f | %d
      mask Display:
      | p={'%f\r\n'; '%d\r\n'; '%f'; '%d'};
      | disp(['sprintf: ' p{format}])

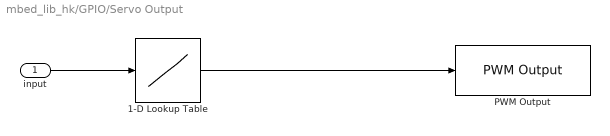
== system mbed_lib_hk/GPIO/Servo Output ==
  input : Inport
  1-D Lookup Table : Lookup_n-D  NumberOfTableDimensions=1  BreakpointsForDimension1=[0 1]  Table=[PW_min PW_max]/20  ExtrapMethod=Clip  UseLastTableValue=on  InternalRulePriority=Speed  RndMeth=Simplest  InputSameDT=on
  PWM Output : mbed_lib/GPIO/PWM Output  SParameter1=A  SParameter2=0  SParameter3=20000  SampleTime=-1
  wires:
  input/1 -> 1-D Lookup Table/1
  1-D Lookup Table/1 -> PWM Output/1

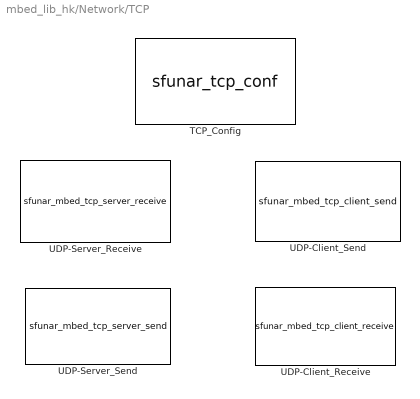
== system mbed_lib_hk/Network/TCP ==
  TCP_Config : S-Function  FunctionName=sfunar_tcp_conf  Parameters=ip_addr, sub_mask, gateway  mask{ip_addr='127.0.0.1', sub_mask='255.255.255.0', gateway='0.0.0.0', SampleTime=-1, DEFAULT_UDP_RECVMBOX_SIZE=8, TCPIP_THREAD_STACKSIZE=1024, TCPIP_THREAD_PRIO=Normal, PBUF_POOL_SIZE=5, TCP_MSS=1460}
      mask prompts: ip_addr "IP-Address"; sub_mask "Sub-Netmask"; SampleTime "Sample time (-1 for inherited):"; DEFAULT_UDP_RECVMBOX_SIZE "TCP Receive M-Box size"; TCPIP_THREAD_STACKSIZE "TCP/IP Thread Stacksize"; TCPIP_THREAD_PRIO "TCP/IP Thread Prio"; PBUF_POOL_SIZE "PBuf Pool Size"; TCP_MSS "TCP Maximun Segment Size"
      mask init:
      | ip = get_param(gcbh,'ip_addr');
      | subm = get_param(gcbh,'sub_mask');
      | MaskDisplay = ['disp(''TCP\nConfiguration\nIP: ' ip(2:end-1) ...
      |                 '\nSub-M.: ' subm(2:end-1) ''');'];
      | set_param(gcbh, 'MaskDisplay', MaskDisplay);
      settings: CopyFcn=|
      | fid = fopen('lwipopts.h','r+t');
      | lwipopts = textscan(fid,'%s','delimiter','\n');
      settings: DestroyFcn=|
      | try
      | fclose(fid);
      | catch ME
      | end
      | disp('Destroy')
      mask Callback DEFAULT_UDP_RECVMBOX_SIZE:
      | try
      | pos_ti_th_ss = find(~cellfun('isempty',strfind(lwipopts{1,1},'DEFAULT_UDP_RECVMBOX_SIZE')));
      | lwipopts{1,1}{pos_ti_th_ss(1)} = ...
      |     sprintf('#define DEFAULT_UDP_RECVMBOX_SIZE\t%d',...
      |             get_param(gcb,'TCPIP_THREAD_STACKSIZE'));
      | 
      | for row = 1:length(lwipopts{1,1})
      |   fprintf(fid, '%s\n', lwipopts{1,1}{row});
      | end
      | 
      | catch exeption
      | end
      mask Callback TCPIP_THREAD_STACKSIZE:
      | try
      | pos_ti_th_ss = find(~cellfun('isempty',strfind(lwipopts{1,1},'TCPIP_THREAD_STACKSIZE')));
      | lwipopts{1,1}{pos_ti_th_ss(1)} = ...
      |     sprintf('#define TCPIP_THREAD_STACKSIZE\t%d',...
      |             get_param(gcb,'TCPIP_THREAD_STACKSIZE'));
      | 
      | for row = 1:length(lwipopts{1,1})
      |   fprintf(fid, '%s\n', lwipopts{1,1}{row});
      | end
      | 
      | catch exeption
      | end
      mask TypeOptions TCPIP_THREAD_PRIO: Idle | Low | Below Normal | Normal | Above Normal | High | Realtime
      mask Callback PBUF_POOL_SIZE:
      | try
      | pos_ti_th_ss = find(~cellfun('isempty',strfind(lwipopts{1,1},'PBUF_POOL_SIZE')));
      | lwipopts{1,1}{pos_ti_th_ss(1)} = ...
      |     sprintf('#define PBUF_POOL_SIZE\t%d',...
      |             get_param(gcb,'TCPIP_THREAD_STACKSIZE'));
      | 
      | for row = 1:length(lwipopts{1,1})
      |   fprintf(fid, '%s\n', lwipopts{1,1}{row});
      | end
      | 
      | catch exeption
      | end
      mask Callback TCP_MSS:
      | try
      | pos_ti_th_ss = find(~cellfun('isempty',strfind(lwipopts{1,1},'TCP_MSS')));
      | lwipopts{1,1}{pos_ti_th_ss(1)} = ...
      |     sprintf('#define TCP_MSS\t%d',...
      |             get_param(gcb,'TCPIP_THREAD_STACKSIZE'));
      | 
      | for row = 1:length(lwipopts{1,1})
      |   fprintf(fid, '%s\n', lwipopts{1,1}{row});
      | end
      | 
      | catch exeption
      | end
      mask Display: disp('TCP\nConfiguration\nIP: 127.0.0.1\nSub-M.: 255.255.255.0');
  UDP-Client_Receive : S-Function  FunctionName=sfunar_mbed_tcp_client_receive  Parameters=sock_ID, caOutputPorts, SampleTime  mask{sock_ID=2, caOutputPorts={'uint8' 'uint16'}, SampleTime=0}
      mask prompts: sock_ID "Socket ID:"; caOutputPorts "Output port data types (cell array):"; SampleTime "Sample time (-1 for inherited):"
      mask init:
      | sock_ID = get_param(gcbh,'sock_ID');
      | MaskDisplay = ['disp(''TCP-Client\nReceive\nId: ' num2str(sock_ID) ''');'];
      | set_param(gcb, 'MaskDisplay', MaskDisplay);
      mask TypeOptions sock_ID: 1 | 2 | 3 | 4 | 5 | 6 | 7 | 8
      mask Display: disp('TCP-Client\nReceive\nId: 2');
  UDP-Client_Send : S-Function  FunctionName=sfunar_mbed_tcp_client_send  Parameters=sock_ID, des_IP, des_port, caInputPorts, SampleTime, nBufferBytes  mask{sock_ID=2, des_IP='192.168.0.50', des_port=5001, caInputPorts={'uint8' 'uint32' 'uint16'}, SampleTime=0, nBufferBytes=0}
      mask prompts: sock_ID "Socket ID:"; des_IP "Destination IP address:"; des_port "Destination Port:"; caInputPorts "Input port (unpacked) data types (cell array):"; SampleTime "Sample time (-1 for inherited):"
      mask init:
      | desip = get_param(gcbh,'des_ip');
      | desp = get_param(gcbh,'des_port');
      | sock_ID = get_param(gcbh,'sock_ID');
      | MaskDisplay = ['disp(''TCP-Client\nSend\nId: ' num2str(sock_ID)...
      |                 '\n Dest.: ' desip(2:end-1) ':' desp ''');'];
      | set_param(gcb, 'MaskDisplay', MaskDisplay);
      mask TypeOptions sock_ID: 1 | 2 | 3 | 4 | 5 | 6 | 7 | 8
      mask Display: disp('TCP-Client\nSend\nId: 2\n Dest.: 192.168.0.50:5001');
  UDP-Server_Receive : S-Function  FunctionName=sfunar_mbed_tcp_server_receive  Parameters=sock_ID, src_port, caOutputPorts, SampleTime  mask{sock_ID=1, src_port=5001, caOutputPorts={'uint8' 'uint16' 'uint32'}, SampleTime=0}
      mask prompts: sock_ID "Socket ID:"; src_port "Source Port:"; caOutputPorts "Output port data types (cell array):"; SampleTime "Sample time (-1 for inherited):"
      mask init:
      | desp = get_param(gcbh,'src_port');
      | sock_ID = get_param(gcbh,'sock_ID');
      | MaskDisplay = ['disp(''TCP-Server\nReceive\nId: ' num2str(sock_ID)...
      |                 '\nSrv.- Port: ' desp ''');'];
      | set_param(gcb, 'MaskDisplay', MaskDisplay);
      mask TypeOptions sock_ID: 1 | 2 | 3 | 4 | 5 | 6 | 7 | 8
      mask Display: disp('TCP-Server\nReceive\nId: 1\nSrv.- Port: 5001');
  UDP-Server_Send : S-Function  FunctionName=sfunar_mbed_tcp_server_send  Parameters=sock_ID, des_IP, srv_port, caInputPorts, SampleTime, nBufferBytes  mask{sock_ID=1, des_IP=0, srv_port=5002, caInputPorts={'uint8' 'uint16' 'uint32'}, SampleTime=0, nBufferBytes=0}
      mask prompts: sock_ID "Socket ID:"; des_IP "Destination IP address:"; srv_port "Destination Port:"; caInputPorts "Input port (unpacked) data types (cell array):"; SampleTime "Sample time (-1 for inherited):"
      mask init:
      | %desip = get_param(gcbh,'des_ip');
      | desp = get_param(gcbh,'srv_port');
      | sock_ID = get_param(gcbh,'sock_ID');
      | MaskDisplay = ['disp(''TCP-Server\nSend\nId: ' num2str(sock_ID) ''');'];
      | set_param(gcb, 'MaskDisplay', MaskDisplay);
      mask TypeOptions sock_ID: 1 | 2 | 3 | 4 | 5 | 6 | 7 | 8
      mask Display: disp('TCP-Server\nSend\nId: 1');
